simulink model "Hss_buckboost_ave_20250604"  (R2024b)
settings: Solver=VariableStepAuto  StartTime=0.0  StopTime=0.2  RelTol=1e-3
StartFcn:
  | tic
StopFcn:
  | toc
values from neighbouring files (symbols this model uses):
  Af = mtoeplitz(A)    [HSS_buckboost_ave_20250528.m]    (also in HSS_buckboost_det_20250528.m; param_BuckboostHSS_ave_simulink_20250604.m; param_BuckboostHSS_det_simulink_20250602.m)
  alpha = 5/17    (= 0.294117647059)    [HSS_buckboost_ave_20250528.m]    (also in HSS_buckboost_det_20250528.m; param_BuckboostHSS_ave_simulink_20250604.m; param_BuckboostHSS_det_simulink_20250602.m)
  Bf = mtoeplitz(B)    [HSS_buckboost_ave_20250528.m]    (also in HSS_buckboost_det_20250528.m; param_BuckboostHSS_ave_simulink_20250604.m; param_BuckboostHSS_det_simulink_20250602.m)
  C = 3.55*10^-3    (= 0.00355)    [HSS_buckboost_ave_20250528.m]    (also in HSS_buckboost_det_20250528.m; param_BuckboostHSS_ave_simulink_20250604.m; param_BuckboostHSS_det_simulink_20250602.m)
  Fnom = 50    [HSS_buckboost_ave_20250528.m]    (also in HSS_buckboost_det_20250528.m; param_BuckboostHSS_ave_simulink_20250604.m; param_BuckboostHSS_det_simulink_20250602.m)
  L = length(t)    [HSS_buckboost_ave_20250528.m]    (also in HSS_buckboost_det_20250528.m; param_BuckboostHSS_ave_simulink_20250604.m; param_BuckboostHSS_det_simulink_20250602.m)
  N = 30    [HSS_buckboost_ave_20250528.m]    (also in HSS_buckboost_det_20250528.m; param_BuckboostHSS_ave_simulink_20250604.m; param_BuckboostHSS_det_simulink_20250602.m)
  Nt = blkdiag(Nt,1i*w0*k*I)    [HSS_buckboost_ave_20250528.m]    (also in HSS_buckboost_det_20250528.m; param_BuckboostHSS_ave_simulink_20250604.m; param_BuckboostHSS_det_simulink_20250602.m)
  R = 3.57    [HSS_buckboost_ave_20250528.m]    (also in HSS_buckboost_det_20250528.m; param_BuckboostHSS_ave_simulink_20250604.m; param_BuckboostHSS_det_simulink_20250602.m)
  Ts = 1e-7    (= 1e-07)    [HSS_buckboost_ave_20250528.m]    (also in HSS_buckboost_det_20250528.m; param_BuckboostHSS_ave_simulink_20250604.m; param_BuckboostHSS_det_simulink_20250602.m)
  Uf = [Uf;u]    [HSS_buckboost_ave_20250528.m]    (also in HSS_buckboost_det_20250528.m = u; param_BuckboostHSS_ave_simulink_20250604.m)
  Vin = 12    [HSS_buckboost_ave_20250528.m]    (also in HSS_buckboost_det_20250528.m; param_BuckboostHSS_ave_simulink_20250604.m; param_BuckboostHSS_det_simulink_20250602.m)
libraries: spsMosfetLib x1, sps_lib x1
settings Model: Creator=DELL  LastModifiedBy=ana
settings OptimizationCC: ReuseModelBlockBuffer=off
settings RTWCC: GPUComputeCapability=3.5

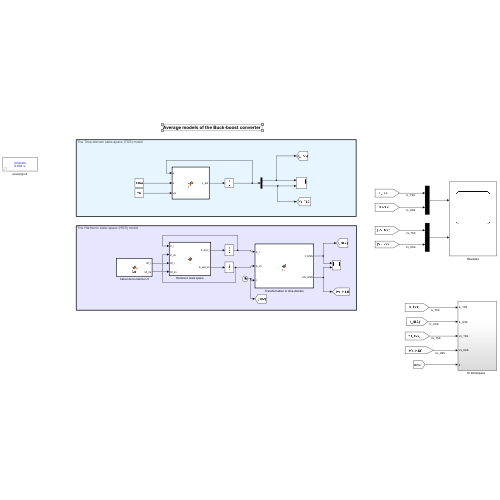
[thumbnail: Simulink's stored preview of the top-level diagram]
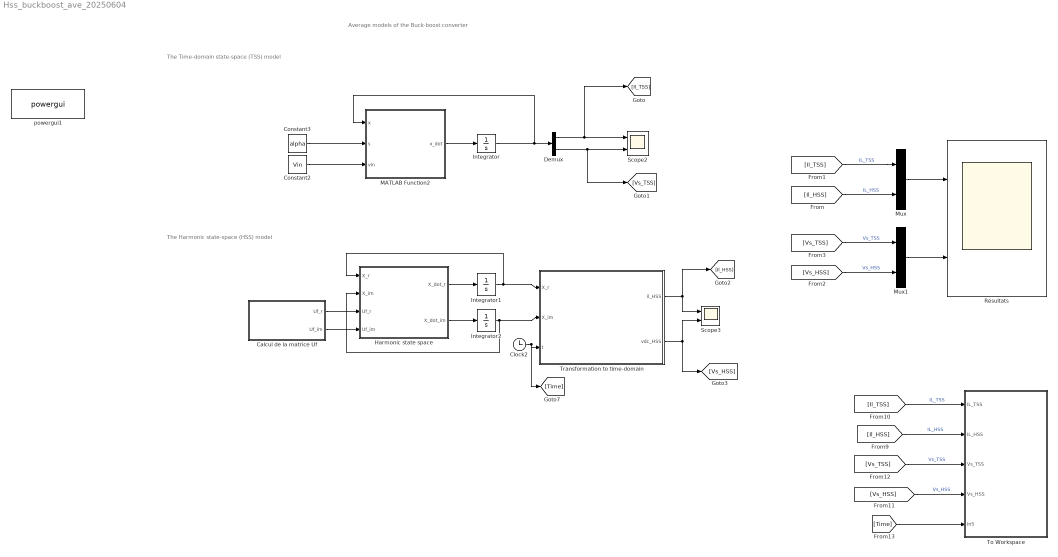
== system Hss_buckboost_ave_20250604 ==
  note: The Harmonic state-space (HSS) model
  note: The Time-domain state-space (TSS) model
  note: Average models of the Buck-boost converter
  Calcul de la matrice Uf : MATLAB Function  TreatAsAtomicUnit=on
  Clock2 : Clock
  Constant2 : Constant  Value=Vin
  Constant3 : Constant  Value=alpha
  Demux : Demux  Outputs=2
  Harmonic state space : MATLAB Function  TreatAsAtomicUnit=on
  Integrator : Integrator
  Integrator1 : Integrator
  Integrator2 : Integrator
  MATLAB Function2 : MATLAB Function  TreatAsAtomicUnit=on
  Mux : Mux  Inputs=2
  Mux1 : Mux  Inputs=2
  Résultats : Scope  NumInputPorts=2
  Scope2 : Scope  NumInputPorts=2
  Scope3 : Scope  NumInputPorts=2
  "To Workspace   " : Subsystem
  Transformation to time-domain : MATLAB Function  TreatAsAtomicUnit=on
  powergui1 : sps_lib/powergui  SimulationMode=Discrete  SampleTime=Ts  frequency=60  Iterations=50  frequencyindice=0  Pbase=100e6  ErrMax=1e-4  UnitsV=kV  UnitsW=MW  buscounter=0  FunctionMessages=off  echomessages=off  EnableUseOfTLC=off  CurrentSourceSwitches=off  DisableSnubberDevices=off  DisableRonSwitches=off  DisableVfSwitches=off  DisplayEquations=off  AutomaticDiscreteSolvers=off  SolverType=Tustin/Backward Euler (TBE)  Interpol=off  ExternalGateDelay=off  methode=off  Ts=0  x0status=blocks  SPID=off  SwTol=0  HookPort=off  NonlinearTolerance=1e-4  nMaxIteration=100  ContinueOnMaxIteration=off  RestoreLinks=warning  ResistiveCurrentMeasurement=off  Frange=[0:2:500]  Ylog=off  Xlog=on  ShowGrid=off  save=off  variable=ZData  structure=ta_loic  ZoomFFT=off  StartTime=0.12  cycles=1  DisplayStyle=2  fundamental=60  FreqAxis=on  MaxFrequency=100000  frequencyindicesteady=1  RmsSteady=1  display=off
  wires:
  Demux/1 -> [Il_TSS], Scope2/1
  MATLAB Function2/1(x_dot) -> Integrator/1
  Demux/2 -> [Vs_TSS], Scope2/2
  Constant2/1 -> MATLAB Function2/3(vin)
  Integrator/1 -> MATLAB Function2/1(x), Demux/1
  Clock2/1 -> [Time], Transformation to time-domain/3(t)
  Calcul de la matrice Uf/1(Uf_r) -> Harmonic state space/3(Uf_r)
  Integrator1/1 -> Transformation to time-domain/1(X_r), Harmonic state space/1(X_r)
  Transformation to time-domain/1(il_HSS) -> [Il_HSS], Scope3/1
  Transformation to time-domain/2(vdc_HSS) -> Scope3/2, [Vs_HSS]
  Harmonic state space/1(X_dot_r) -> Integrator1/1
  Constant3/1 -> MATLAB Function2/2(s)
  [Il_TSS] -> Mux/1  "IL_TSS"
  [Il_HSS] -> Mux/2  "IL_HSS"
  Mux/1 -> Résultats/1
  Mux1/1 -> Résultats/2
  [Vs_TSS] -> Mux1/1  "Vs_TSS"
  [Vs_HSS] -> Mux1/2  "Vs_HSS"
  [Vs_HSS] -> "To Workspace   "/4(Vs_HSS)  "Vs_HSS"
  [Il_TSS] -> "To Workspace   "/1(IL_TSS)  "IL_TSS"
  [Vs_TSS] -> "To Workspace   "/3(Vs_TSS)  "Vs_TSS"
  [Il_HSS] -> "To Workspace   "/2(IL_HSS)  "IL_HSS"
  [Time] -> "To Workspace   "/5(In5)
  Calcul de la matrice Uf/2(Uf_im) -> Harmonic state space/4(Uf_im)
  Harmonic state space/2(X_dot_im) -> Integrator2/1
  Integrator2/1 -> Harmonic state space/2(X_im), Transformation to time-domain/2(X_im)

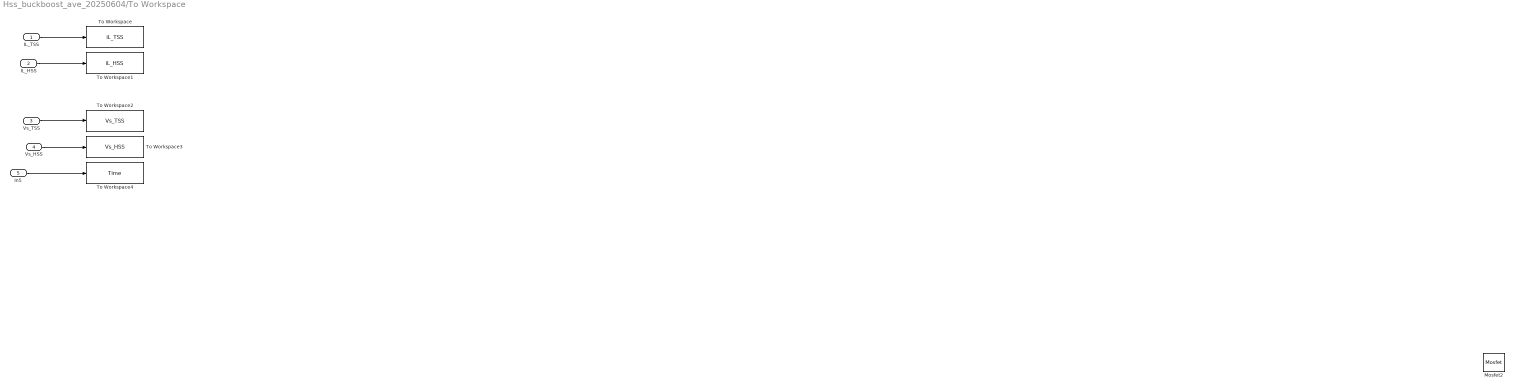
== system Hss_buckboost_ave_20250604/To Workspace    ==
  IL_TSS : Inport
  IL_HSS : Inport  Port=2
  Vs_TSS : Inport  Port=3
  Vs_HSS : Inport  Port=4
  In5 : Inport  Port=5
  Mosfet2 : spsMosfetLib/Mosfet  Ron=0.1  Lon=0  Rd=0.01  Vfd=0  IC=0  Rs=1e5  Cs=inf  Measurements=on
  To Workspace : ToWorkspace  VariableName=iL_TSS  SampleTime=-1
  To Workspace1 : ToWorkspace  VariableName=iL_HSS  SampleTime=-1
  To Workspace2 : ToWorkspace  VariableName=Vs_TSS  SampleTime=-1
  To Workspace3 : ToWorkspace  VariableName=Vs_HSS  SampleTime=-1
  To Workspace4 : ToWorkspace  VariableName=Time  SampleTime=-1
  wires:
  IL_TSS/1 -> To Workspace/1
  In5/1 -> To Workspace4/1
  IL_HSS/1 -> To Workspace1/1
  Vs_HSS/1 -> To Workspace3/1
  Vs_TSS/1 -> To Workspace2/1

== matlab function Hss_buckboost_ave_20250604/Transformation to time-domain ==
  data: X_r input size=[(2*N+1)*2,1]; X_im input; t input; il_HSS output; vdc_HSS output; N parameter; Fnom parameter
function [il_HSS,vdc_HSS] = fcn(X_r,X_im,t,N, Fnom)

w0 = 2*pi*Fnom;

Xss = X_r+1i*X_im;

%% Restitution of vectors from Xss
Il = zeros(2*N+1,1);
Vs = zeros(2*N+1,1);
v = [Il,Vs];     % Matrix composed by the Fourier coefficients
v_r=[Il,Vs];
v_i=[Il,Vs];

for i = 1:size(v,2)
    j = i;
    k = 1;                 
    while j <= (2*N+1)*2
        v_r(k,i) = real(Xss(j));
        v_i(k,i) = imag(Xss(j));
        j = j+2;
        k = k+1;
    end
end

v=v_r+1i*v_i;
gamma = 0;

for k = -N:N
    if k==-N
        gamma = exp(w0*k*1i*t);
    else
        gamma = [gamma, exp(w0*k*1i*t)];
    end
end

il_HSS = real(gamma*v(:,1)); % il(t) = sum_k=-N:N( Il_k . exp(+w0*k*1i*t) )
vdc_HSS = real(gamma*v(:,2)); % Vs(t) = sum_k=-N:N( Vs_k . exp(+w0*k*1i*t) )

== matlab function Hss_buckboost_ave_20250604/Calcul de la matrice Uf ==
  data: Uf_r output size=[(2*N+1),1]; R parameter; C parameter; L parameter; N parameter; Uf parameter; Uf_im output
function [Uf_r , Uf_im] = fcn(R, C, L, N, Uf)

Uf_r = real(Uf);
Uf_im = imag(Uf);

== matlab function Hss_buckboost_ave_20250604/MATLAB Function2 ==
  data: x input size=[2,1]; x_dot output; s input; vin input; L parameter; C parameter; R parameter

function x_dot  = fcn(x, s, vin,L, C, R)

il = x(1);
vs = x(2);

sw =s;

il_dot = ((sw/L)*vin+((1-sw)/L)*vs);

vs_dot = (((sw-1)/C)*il+(-1/(R*C))*vs);

x_dot = [il_dot;vs_dot];

== matlab function Hss_buckboost_ave_20250604/Harmonic state space ==
  settings: updateMethod=CONTINUOUS  sampleTime=Ts
  data: X_r input size=[(2*N+1)*2,1]; X_im input; Uf_r input size=[(2*N+1),1]; Uf_im input; X_dot_r output size=[(2*N+1)*2,1]; Af parameter; Bf parameter; Nt parameter; X_dot_im output
function [X_dot_r, X_dot_im]   = fcn(X_r,X_im,Uf_r, Uf_im, Af,Bf,Nt)
X = X_r+1i*X_im;

Uf = Uf_r+1i*Uf_im;
X_dot = (Af-Nt)*X+Bf*Uf;

X_dot_r = real(X_dot);
X_dot_im = imag(X_dot);
